simulink model "DevChallengeETRS"  (R2025b)
settings: Solver=ode3  StartTime=0.0  StopTime=10.0  FixedStep=0.001  RelTol=1e-3
settings Model: Creator=George  LastModifiedBy=Hao Yan
settings RTWCC: GPUComputeCapability=3.5

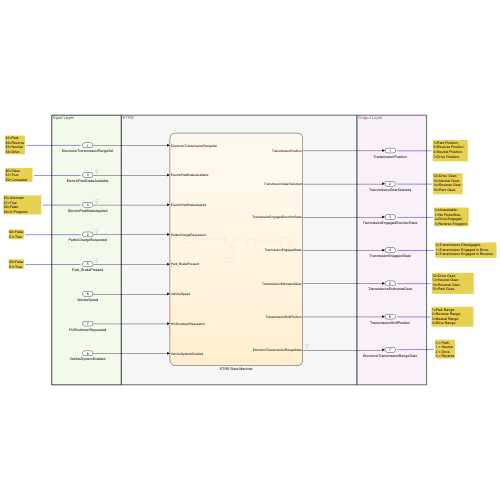
[thumbnail: Simulink's stored preview of the top-level diagram]
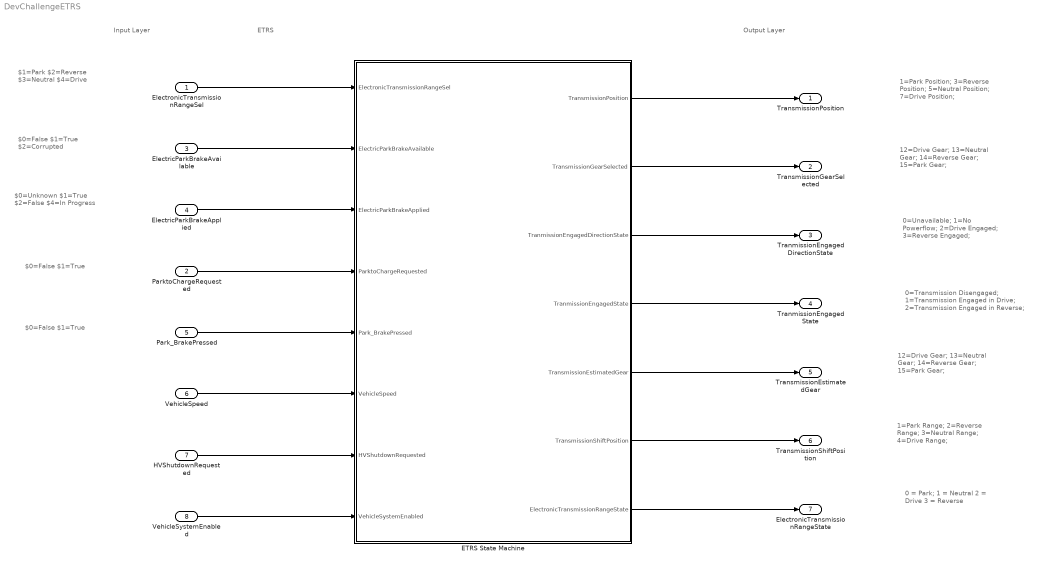
== system DevChallengeETRS ==
  note: 0 = Park;
      | 1 = Neutral
      | 2 = Drive
      | 3 = Reverse
  note: $1=Park
      | $2=Reverse
      | $3=Neutral
      | $4=Drive
  note: 1=Park Position;
      | 3=Reverse Position;
      | 5=Neutral Position;
      | 7=Drive Position;
  note: 0=Unavailable;
      | 1=No Powerflow;
      | 2=Drive Engaged;
      | 3=Reverse Engaged;
  note: 12=Drive Gear;
      | 13=Neutral Gear;
      | 14=Reverse Gear;
      | 15=Park Gear;
  note: ETRS
  note: 1=Park Range;
      | 2=Reverse Range;
      | 3=Neutral Range;
      | 4=Drive Range;
  note: $0=Unknown
      | $1=True
      | $2=False
      | $4=In Progress
  note: 0=Transmission Disengaged;
      | 1=Transmission Engaged in Drive;
      | 2=Transmission Engaged in Reverse;
  note: $0=False
      | $1=True
  note: 12=Drive Gear;
      | 13=Neutral Gear;
      | 14=Reverse Gear;
      | 15=Park Gear;
  note: $0=False
      | $1=True
      | $2=Corrupted
  note: $0=False
      | $1=True
  note: Input Layer
  note: Output Layer
  ElectronicTransmissionRangeSel : Inport
  ParktoChargeRequested : Inport  Port=2
  ElectricParkBrakeAvailable : Inport  Port=3
  ElectricParkBrakeApplied : Inport  Port=4
  Park_BrakePressed : Inport  Port=5
  VehicleSpeed : Inport  Port=6
  HVShutdownRequested : Inport  Port=7
  VehicleSystemEnabled : Inport  Port=8
  ETRS State Machine : Stateflow chart  TreatAsAtomicUnit=on
  TransmissionPosition : Outport
  TransmissionGearSelected : Outport  Port=2
  TranmissionEngagedDirectionState : Outport  Port=3
  TranmissionEngagedState : Outport  Port=4
  TransmissionEstimatedGear : Outport  Port=5
  TransmissionShiftPosition : Outport  Port=6
  ElectronicTransmissionRangeState : Outport  Port=7
  wires:
  ParktoChargeRequested/1 -> ETRS State Machine/4(ParktoChargeRequested)
  ElectronicTransmissionRangeSel/1 -> ETRS State Machine/1(ElectronicTransmissionRangeSel)
  ETRS State Machine/4(TranmissionEngagedState) -> TranmissionEngagedState/1
  ETRS State Machine/2(TransmissionGearSelected) -> TransmissionGearSelected/1
  ElectricParkBrakeApplied/1 -> ETRS State Machine/3(ElectricParkBrakeApplied)
  ETRS State Machine/5(TransmissionEstimatedGear) -> TransmissionEstimatedGear/1
  ETRS State Machine/6(TransmissionShiftPosition) -> TransmissionShiftPosition/1
  ETRS State Machine/1(TransmissionPosition) -> TransmissionPosition/1
  ElectricParkBrakeAvailable/1 -> ETRS State Machine/2(ElectricParkBrakeAvailable)
  ETRS State Machine/3(TranmissionEngagedDirectionState) -> TranmissionEngagedDirectionState/1
  ETRS State Machine/7(ElectronicTransmissionRangeState) -> ElectronicTransmissionRangeState/1
  Park_BrakePressed/1 -> ETRS State Machine/5(Park_BrakePressed)
  VehicleSpeed/1 -> ETRS State Machine/6(VehicleSpeed)
  HVShutdownRequested/1 -> ETRS State Machine/7(HVShutdownRequested)
  VehicleSystemEnabled/1 -> ETRS State Machine/8(VehicleSystemEnabled)

== stateflow chart DevChallengeETRS/ETRS State Machine ==
  state Park
    entry:
    TransmissionPosition = 1;
    TransmissionShiftPosition = 1;
    TransmissionEstimatedGear = 15;
    TransmissionGearSelected = 15;
    TranmissionEngagedState = 0;
    TranmissionEngagedDirectionState = 1;
    ElectronicTransmissionRangeState = 0;
  state Neutral
    entry:
    TransmissionPosition = 5;
    TransmissionShiftPosition = 3;
    TransmissionEstimatedGear = 13;
    TransmissionGearSelected = 13;
    TranmissionEngagedState = 0;
    TranmissionEngagedDirectionState = 1;
    ElectronicTransmissionRangeState = 1;
  state Drive
    entry:
    TransmissionPosition = 7;
    TransmissionShiftPosition = 4;
    TransmissionEstimatedGear = 12;
    TransmissionGearSelected = 12;
    TranmissionEngagedState = 1;
    TranmissionEngagedDirectionState = 2;
    ElectronicTransmissionRangeState = 2;
  state Neutral_Intermediate_Drive
    entry:
    TransmissionPosition = 5;
    TransmissionShiftPosition = 3;
    TransmissionEstimatedGear = 13;
    TransmissionGearSelected = 13;
    TranmissionEngagedState = 0;
    TranmissionEngagedDirectionState = 1;
    ElectronicTransmissionRangeState = 4
  state Neutral_Intermediate_Reverse
    entry:
    TransmissionPosition = 5;
    TransmissionShiftPosition = 3;
    TransmissionEstimatedGear = 13;
    TransmissionGearSelected = 13;
    TranmissionEngagedState = 0;
    TranmissionEngagedDirectionState = 1;
    ElectronicTransmissionRangeState = 5;
  state Reverse
    entry:
    TransmissionPosition = 3;
    TransmissionShiftPosition = 2;
    TransmissionEstimatedGear = 14;
    TransmissionGearSelected = 14;
    TranmissionEngagedState = 2;
    TranmissionEngagedDirectionState = 3;
    ElectronicTransmissionRangeState = 3;
  (default) -> Park
  Neutral -> Park [order 2] : [(ElectronicTransmissionRangeSel == 1 || ParktoChargeRequested == 1) && ElectricParkBrakeAvailable == 1 && ...
      | VehicleSpeed < 0.5 && ElectricParkBrakeApplied == 1]
  Neutral -> Drive [order 3] : [ElectronicTransmissionRangeSel == 4 && ElectricParkBrakeApplied == 2 && VehicleSystemEnabled == 1]
  Park -> Neutral : [((ElectronicTransmissionRangeSel ~= 1 && ElectronicTransmissionRangeSel ~= 0) || (ElectricParkBrakeApplied == 2 || ElectricParkBrakeApplied == 4))...
      | && ParktoChargeRequested == 0 && VehicleSpeed < 0.5 && Park_BrakePressed == 1]
  Neutral_Intermediate_Drive -> Neutral [order 1] : [VehicleSpeed < 0.5]
  Drive -> Neutral_Intermediate_Drive : [((ElectronicTransmissionRangeSel ~= 4 || ParktoChargeRequested == 1 || ElectricParkBrakeApplied == 1) || HVShutdownRequested == 1)]
  Neutral -> Reverse [order 1] : [ElectronicTransmissionRangeSel == 2  && ElectricParkBrakeApplied == 2 && VehicleSystemEnabled == 1]
  Neutral_Intermediate_Reverse -> Neutral [order 1] : [VehicleSpeed < 0.5]
  Neutral_Intermediate_Drive -> Drive [order 2] : [ElectronicTransmissionRangeSel == 4 && ParktoChargeRequested == 0 && ElectricParkBrakeApplied == 2 && ...
      |   VehicleSystemEnabled == 1]
  Neutral_Intermediate_Reverse -> Reverse [order 2] : [ElectronicTransmissionRangeSel == 2 && ParktoChargeRequested == 0 && ElectricParkBrakeApplied == 2 ...
      |  && VehicleSystemEnabled == 1]
  Reverse -> Neutral_Intermediate_Reverse : [(ElectronicTransmissionRangeSel ~= 2 || ParktoChargeRequested == 1 || ElectricParkBrakeApplied == 1) || HVShutdownRequested == 1]
  data: ElectronicTransmissionRangeSel input; ElectricParkBrakeAvailable input; ElectricParkBrakeApplied input; TransmissionPosition output; TransmissionGearSelected output; TranmissionEngagedDirectionState output; TranmissionEngagedState output; TransmissionEstimatedGear output; TransmissionShiftPosition output; ParktoChargeRequested input; Park_BrakePressed input boolean; VehicleSpeed input; HVShutdownRequested input; VehicleSystemEnabled input; ElectronicTransmissionRangeState output
